simulink model "sim"  (R2024a)
settings: Solver=VariableStepAuto  StartTime=0.0  StopTime=500  RelTol=1e-3
undefined symbols (not defined in the file): K1, K2, K3, Ke1, Ke2, Ke3, Kr
settings Model: Creator=grabo  LastModifiedBy=grabo

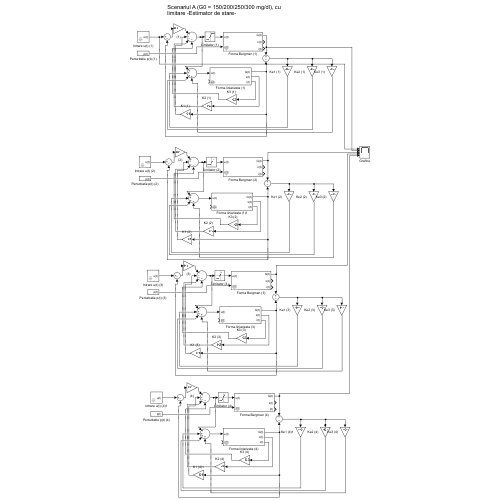
[thumbnail: Simulink's stored preview of the top-level diagram]
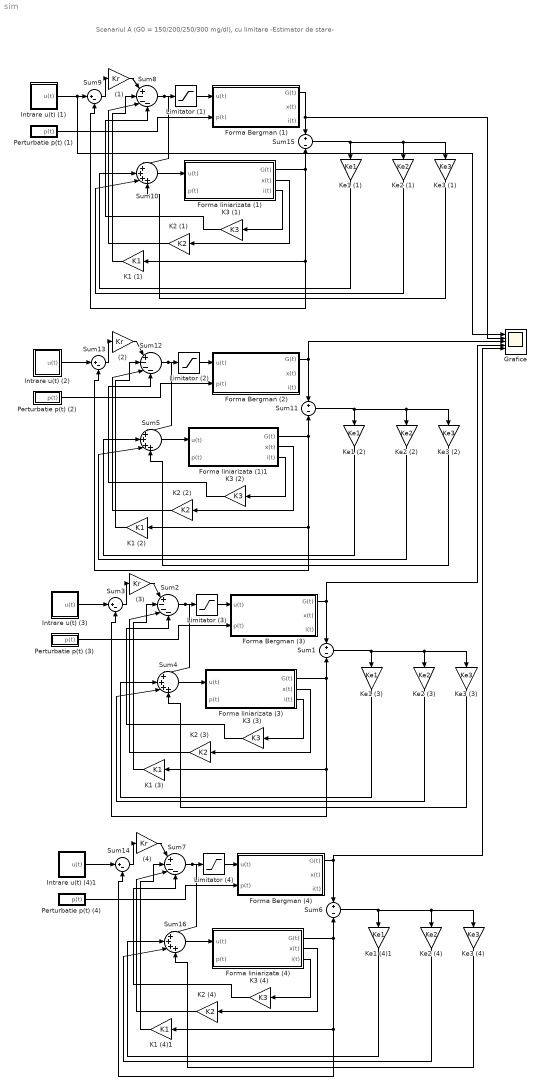
== system sim ==
  note: Scenariul A (G0 = 150/200/250/300 mg/dl), cu limitare -Estimator de stare-
  (1) : Gain  Gain=Kr
  (2) : Gain  Gain=Kr
  (3) : Gain  Gain=Kr
  (4) : Gain  Gain=Kr
  Forma Bergman (1) : Subsystem  mask{V=120, Gb=80, p1=0.019, p2=0.021, p3=10.19*10^(-6), n=0.177, G0=150}
      mask prompts: V "V ="; Gb "Gb ="; p1 "p1 ="; p2 "p2 ="; p3 "p3 ="; n "n ="; G0 "G0 ="
  Forma Bergman (2) : Subsystem  mask{V=120, Gb=80, p1=0.019, p2=0.021, p3=10.19*10^(-6), n=0.177, G0=200}
      mask prompts: V "V ="; Gb "Gb ="; p1 "p1 ="; p2 "p2 ="; p3 "p3 ="; n "n ="; G0 "G0 ="
  Forma Bergman (3) : Subsystem  mask{V=120, Gb=80, p1=0.019, p2=0.021, p3=10.19*10^(-6), n=0.177, G0=250}
      mask prompts: V "V ="; Gb "Gb ="; p1 "p1 ="; p2 "p2 ="; p3 "p3 ="; n "n ="; G0 "G0 ="
  Forma Bergman (4) : Subsystem  mask{V=120, Gb=80, p1=0.019, p2=0.021, p3=10.19*10^(-6), n=0.177, G0=300}
      mask prompts: V "V ="; Gb "Gb ="; p1 "p1 ="; p2 "p2 ="; p3 "p3 ="; n "n ="; G0 "G0 ="
  Forma liniarizata (1) : Subsystem  mask{V=120, Ag=0.8, tgM=40, Xb=0.0054, Gb=80, p1=0.019, p2=0.021, p3=10.19*10^(-6), n=0.177, G0=150}
      mask prompts: V "V ="; Ag "Ag ="; tgM "tgM ="; Xb "Xb ="; Gb "Gb ="; p1 "p1 ="; p2 "p2 ="; p3 "p3 ="; n "n ="; G0 "G0 ="
  Forma liniarizata (1)1 : Subsystem  mask{V=120, Ag=0.8, tgM=40, Xb=0.0054, Gb=80, p1=0.019, p2=0.021, p3=10.19*10^(-6), n=0.177, G0=200}
      mask prompts: V "V ="; Ag "Ag ="; tgM "tgM ="; Xb "Xb ="; Gb "Gb ="; p1 "p1 ="; p2 "p2 ="; p3 "p3 ="; n "n ="; G0 "G0 ="
  Forma liniarizata (3) : Subsystem  mask{V=120, Ag=0.8, tgM=40, Xb=0.0054, Gb=80, p1=0.019, p2=0.021, p3=10.19*10^(-6), n=0.177, G0=250}
      mask prompts: V "V ="; Ag "Ag ="; tgM "tgM ="; Xb "Xb ="; Gb "Gb ="; p1 "p1 ="; p2 "p2 ="; p3 "p3 ="; n "n ="; G0 "G0 ="
  Forma liniarizata (4) : Subsystem  mask{V=120, Ag=0.8, tgM=40, Xb=0.0054, Gb=80, p1=0.019, p2=0.021, p3=10.19*10^(-6), n=0.177, G0=300}
      mask prompts: V "V ="; Ag "Ag ="; tgM "tgM ="; Xb "Xb ="; Gb "Gb ="; p1 "p1 ="; p2 "p2 ="; p3 "p3 ="; n "n ="; G0 "G0 ="
  Grafice : Scope  NumInputPorts=5
  Intrare u(t) (1) : Subsystem  mask{With_u=1, Gref=80}
      mask prompts: With_u "With_u ="; Gref "Gref ="
  Intrare u(t) (2) : Subsystem  mask{With_u=1, Gref=80}
      mask prompts: With_u "With_u ="; Gref "Gref ="
  Intrare u(t) (3) : Subsystem  mask{With_u=1, Gref=80}
      mask prompts: With_u "With_u ="; Gref "Gref ="
  Intrare u(t) (4)1 : Subsystem  mask{With_u=1, Gref=80}
      mask prompts: With_u "With_u ="; Gref "Gref ="
  K1 (1) : Gain  Gain=K1
  K1 (2) : Gain  Gain=K1
  K1 (3) : Gain  Gain=K1
  K1 (4)1 : Gain  Gain=K1
  K2 (1) : Gain  Gain=K2
  K2 (2) : Gain  Gain=K2
  K2 (3) : Gain  Gain=K2
  K2 (4) : Gain  Gain=K2
  K3 (1) : Gain  Gain=K3
  K3 (2) : Gain  Gain=K3
  K3 (3) : Gain  Gain=K3
  K3 (4) : Gain  Gain=K3
  Ke1 (1) : Gain  Gain=Ke1
  Ke1 (2) : Gain  Gain=Ke1
  Ke1 (3) : Gain  Gain=Ke1
  Ke1 (4)1 : Gain  Gain=Ke1
  Ke2 (1) : Gain  Gain=Ke2
  Ke2 (2) : Gain  Gain=Ke2
  Ke2 (3) : Gain  Gain=Ke2
  Ke2 (4) : Gain  Gain=Ke2
  Ke3 (1) : Gain  Gain=Ke3
  Ke3 (2) : Gain  Gain=Ke3
  Ke3 (3) : Gain  Gain=Ke3
  Ke3 (4) : Gain  Gain=Ke3
  Limitator (1) : Saturate  UpperLimit=500  LowerLimit=0
  Limitator (2) : Saturate  UpperLimit=500  LowerLimit=0
  Limitator (3) : Saturate  UpperLimit=500  LowerLimit=0
  Limitator (4) : Saturate  UpperLimit=500  LowerLimit=0
  Perturbatie p(t) (1) : Subsystem  mask{Dg=10*10^3, Ag=0.8, tgM=40, With_p=0}
      mask prompts: Dg "Dg ="; Ag "Ag ="; tgM "tgM ="; With_p "With_p ="
  Perturbatie p(t) (2) : Subsystem  mask{Dg=10*10^3, Ag=0.8, tgM=40, With_p=0}
      mask prompts: Dg "Dg ="; Ag "Ag ="; tgM "tgM ="; With_p "With_p ="
  Perturbatie p(t) (3) : Subsystem  mask{Dg=10*10^3, Ag=0.8, tgM=40, With_p=0}
      mask prompts: Dg "Dg ="; Ag "Ag ="; tgM "tgM ="; With_p "With_p ="
  Perturbatie p(t) (4) : Subsystem  mask{Dg=10*10^3, Ag=0.8, tgM=40, With_p=0}
      mask prompts: Dg "Dg ="; Ag "Ag ="; tgM "tgM ="; With_p "With_p ="
  Sum{1,6,11,15} (4 alike) : Sum  Inputs=+|-
  Sum{4..5,10,16} (4 alike) : Sum  Inputs=|++++
  Sum{2,7..8,12} (4 alike) : Sum  Inputs=|+---
  Sum{3,9,13..14} (4 alike) : Sum  Inputs=|+-
  wires:
  Intrare u(t) (1)/1(u(t)) -> Grafice/1, Sum9/1
  Sum8/1 -> Sum10/1, Limitator (1)/1
  Forma liniarizata (1)/1(G(t)) -> Sum15/2, K1 (1)/1, Sum9/2
  Sum10/1 -> Forma liniarizata (1)/1(u(t))
  Forma liniarizata (1)/2(x(t)) -> K2 (1)/1
  Forma liniarizata (1)/3(i(t)) -> K3 (1)/1
  K1 (1)/1 -> Sum8/2
  K2 (1)/1 -> Sum8/3
  K3 (1)/1 -> Sum8/4
  Sum15/1 -> Ke3 (1)/1, Ke2 (1)/1, Ke1 (1)/1
  Ke1 (1)/1 -> Sum10/2
  Ke2 (1)/1 -> Sum10/3
  Ke3 (1)/1 -> Sum10/4
  Ke1 (2)/1 -> Sum5/2
  Intrare u(t) (2)/1(u(t)) -> Sum13/1
  Sum11/1 -> Ke3 (2)/1, Ke2 (2)/1, Ke1 (2)/1
  K1 (2)/1 -> Sum12/2
  K2 (2)/1 -> Sum12/3
  Forma liniarizata (1)1/1(G(t)) -> Sum11/2, K1 (2)/1, Sum13/2
  Sum5/1 -> Forma liniarizata (1)1/1(u(t))
  Sum12/1 -> Sum5/1, Limitator (2)/1
  K3 (2)/1 -> Sum12/4
  Ke3 (2)/1 -> Sum5/4
  Forma Bergman (2)/1(G(t)) -> Grafice/3, Sum11/1
  Forma liniarizata (1)1/2(x(t)) -> K2 (2)/1
  Forma liniarizata (1)1/3(i(t)) -> K3 (2)/1
  Ke2 (2)/1 -> Sum5/3
  (1)/1 -> Sum8/1
  Sum9/1 -> (1)/1
  (2)/1 -> Sum12/1
  Sum13/1 -> (2)/1
  Forma Bergman (1)/1(G(t)) -> Grafice/2, Sum15/1
  Limitator (2)/1 -> Forma Bergman (2)/1(u(t))
  Limitator (1)/1 -> Forma Bergman (1)/1(u(t))
  Perturbatie p(t) (1)/1(p(t)) -> Forma Bergman (1)/2(p(t))
  Perturbatie p(t) (2)/1(p(t)) -> Forma Bergman (2)/2(p(t))
  Perturbatie p(t) (3)/1(p(t)) -> Forma Bergman (3)/2(p(t))
  Limitator (3)/1 -> Forma Bergman (3)/1(u(t))
  Ke1 (3)/1 -> Sum4/2
  Ke2 (3)/1 -> Sum4/3
  K3 (3)/1 -> Sum2/4
  Forma liniarizata (3)/1(G(t)) -> Sum1/2, K1 (3)/1, Sum3/2
  Forma Bergman (3)/1(G(t)) -> Grafice/4, Sum1/1
  Ke3 (3)/1 -> Sum4/4
  Sum2/1 -> Sum4/1, Limitator (3)/1
  Forma liniarizata (3)/3(i(t)) -> K3 (3)/1
  Sum4/1 -> Forma liniarizata (3)/1(u(t))
  K2 (3)/1 -> Sum2/3
  K1 (3)/1 -> Sum2/2
  (3)/1 -> Sum2/1
  Intrare u(t) (3)/1(u(t)) -> Sum3/1
  Forma liniarizata (3)/2(x(t)) -> K2 (3)/1
  Sum1/1 -> Ke3 (3)/1, Ke2 (3)/1, Ke1 (3)/1
  Sum3/1 -> (3)/1
  Perturbatie p(t) (4)/1(p(t)) -> Forma Bergman (4)/2(p(t))
  Limitator (4)/1 -> Forma Bergman (4)/1(u(t))
  Ke1 (4)1/1 -> Sum16/2
  Ke2 (4)/1 -> Sum16/3
  K3 (4)/1 -> Sum7/4
  Forma liniarizata (4)/1(G(t)) -> Sum6/2, K1 (4)1/1, Sum14/2
  Forma Bergman (4)/1(G(t)) -> Grafice/5, Sum6/1
  Ke3 (4)/1 -> Sum16/4
  Sum7/1 -> Sum16/1, Limitator (4)/1
  Forma liniarizata (4)/3(i(t)) -> K3 (4)/1
  Sum16/1 -> Forma liniarizata (4)/1(u(t))
  K2 (4)/1 -> Sum7/3
  K1 (4)1/1 -> Sum7/2
  (4)/1 -> Sum7/1
  Intrare u(t) (4)1/1(u(t)) -> Sum14/1
  Forma liniarizata (4)/2(x(t)) -> K2 (4)/1
  Sum6/1 -> Ke3 (4)/1, Ke2 (4)/1, Ke1 (4)1/1
  Sum14/1 -> (4)/1

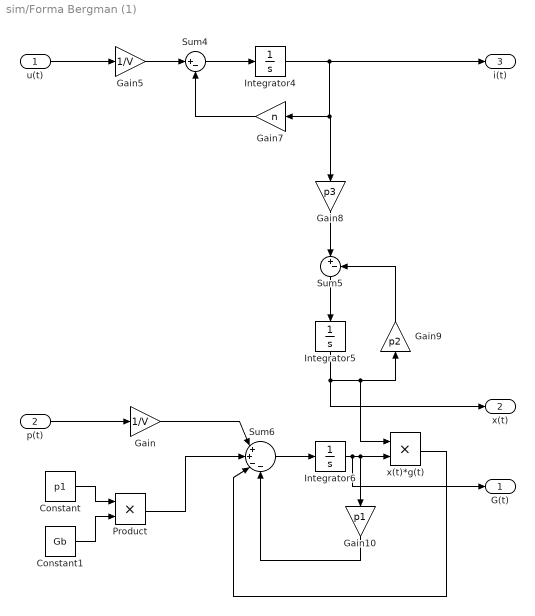
== system sim/Forma Bergman (1) ==
  u(t) : Inport
  p(t) : Inport  Port=2
  Constant : Constant  Value=p1
  Constant1 : Constant  Value=Gb
  Gain : Gain  Gain=1/V
  Gain10 : Gain  Gain=p1
  Gain5 : Gain  Gain=1/V
  Gain7 : Gain  Gain=n
  Gain8 : Gain  Gain=p3
  Gain9 : Gain  Gain=p2
  Integrator4 : Integrator
  Integrator5 : Integrator
  Integrator6 : Integrator  InitialCondition=G0
  Product : Product
  Sum4 : Sum  Inputs=|+-
  Sum5 : Sum  Inputs=|+-
  Sum6 : Sum  Inputs=|++--
  x(t)*g(t) : Product
  G(t) : Outport
  x(t) : Outport  Port=2
  i(t) : Outport  Port=3
  wires:
  Sum4/1 -> Integrator4/1
  Gain7/1 -> Sum4/2
  Integrator4/1 -> Gain7/1, Gain8/1, i(t)/1
  Gain8/1 -> Sum5/1
  Sum5/1 -> Integrator5/1
  Gain9/1 -> Sum5/2
  Sum6/1 -> Integrator6/1
  Integrator6/1 -> G(t)/1, Gain10/1, x(t)*g(t)/2
  Gain10/1 -> Sum6/4
  x(t)*g(t)/1 -> Sum6/3
  Product/1 -> Sum6/2
  Integrator5/1 -> x(t)/1, x(t)*g(t)/1, Gain9/1
  Gain5/1 -> Sum4/1
  u(t)/1 -> Gain5/1
  p(t)/1 -> Gain/1
  Gain/1 -> Sum6/1
  Constant/1 -> Product/1
  Constant1/1 -> Product/2

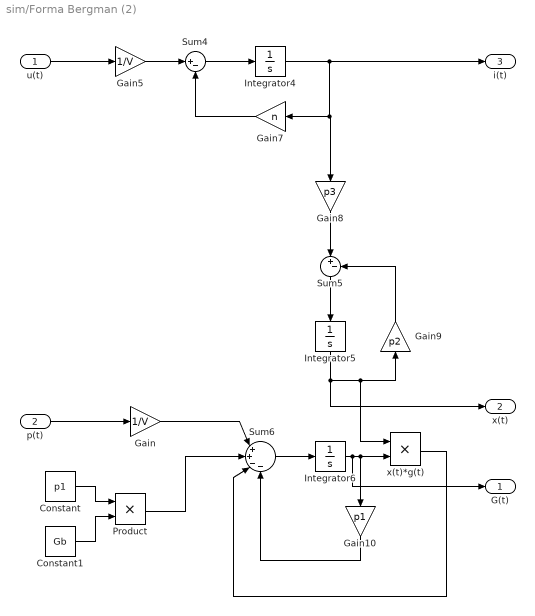
== system sim/Forma Bergman (2) ==
  u(t) : Inport
  p(t) : Inport  Port=2
  Constant : Constant  Value=p1
  Constant1 : Constant  Value=Gb
  Gain : Gain  Gain=1/V
  Gain10 : Gain  Gain=p1
  Gain5 : Gain  Gain=1/V
  Gain7 : Gain  Gain=n
  Gain8 : Gain  Gain=p3
  Gain9 : Gain  Gain=p2
  Integrator4 : Integrator
  Integrator5 : Integrator
  Integrator6 : Integrator  InitialCondition=G0
  Product : Product
  Sum4 : Sum  Inputs=|+-
  Sum5 : Sum  Inputs=|+-
  Sum6 : Sum  Inputs=|++--
  x(t)*g(t) : Product
  G(t) : Outport
  x(t) : Outport  Port=2
  i(t) : Outport  Port=3
  wires:
  Sum4/1 -> Integrator4/1
  Gain7/1 -> Sum4/2
  Integrator4/1 -> Gain7/1, Gain8/1, i(t)/1
  Gain8/1 -> Sum5/1
  Sum5/1 -> Integrator5/1
  Gain9/1 -> Sum5/2
  Sum6/1 -> Integrator6/1
  Integrator6/1 -> G(t)/1, Gain10/1, x(t)*g(t)/2
  Gain10/1 -> Sum6/4
  x(t)*g(t)/1 -> Sum6/3
  Product/1 -> Sum6/2
  Integrator5/1 -> x(t)/1, x(t)*g(t)/1, Gain9/1
  Gain5/1 -> Sum4/1
  u(t)/1 -> Gain5/1
  p(t)/1 -> Gain/1
  Gain/1 -> Sum6/1
  Constant/1 -> Product/1
  Constant1/1 -> Product/2

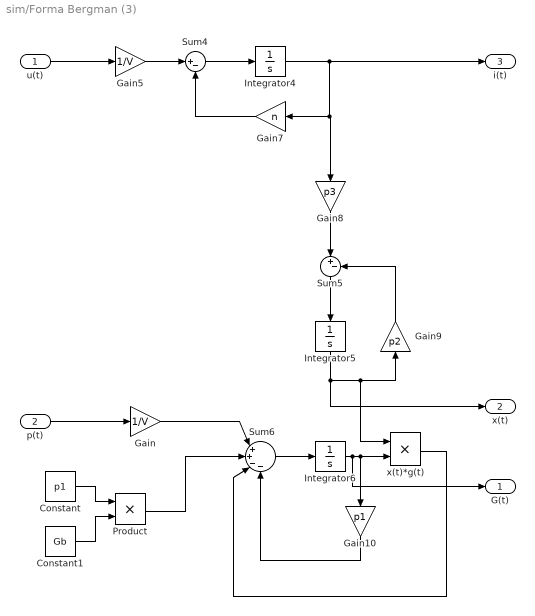
== system sim/Forma Bergman (3) ==
  u(t) : Inport
  p(t) : Inport  Port=2
  Constant : Constant  Value=p1
  Constant1 : Constant  Value=Gb
  Gain : Gain  Gain=1/V
  Gain10 : Gain  Gain=p1
  Gain5 : Gain  Gain=1/V
  Gain7 : Gain  Gain=n
  Gain8 : Gain  Gain=p3
  Gain9 : Gain  Gain=p2
  Integrator4 : Integrator
  Integrator5 : Integrator
  Integrator6 : Integrator  InitialCondition=G0
  Product : Product
  Sum4 : Sum  Inputs=|+-
  Sum5 : Sum  Inputs=|+-
  Sum6 : Sum  Inputs=|++--
  x(t)*g(t) : Product
  G(t) : Outport
  x(t) : Outport  Port=2
  i(t) : Outport  Port=3
  wires:
  Sum4/1 -> Integrator4/1
  Gain7/1 -> Sum4/2
  Integrator4/1 -> Gain7/1, Gain8/1, i(t)/1
  Gain8/1 -> Sum5/1
  Sum5/1 -> Integrator5/1
  Gain9/1 -> Sum5/2
  Sum6/1 -> Integrator6/1
  Integrator6/1 -> G(t)/1, Gain10/1, x(t)*g(t)/2
  Gain10/1 -> Sum6/4
  x(t)*g(t)/1 -> Sum6/3
  Product/1 -> Sum6/2
  Integrator5/1 -> x(t)/1, x(t)*g(t)/1, Gain9/1
  Gain5/1 -> Sum4/1
  u(t)/1 -> Gain5/1
  p(t)/1 -> Gain/1
  Gain/1 -> Sum6/1
  Constant/1 -> Product/1
  Constant1/1 -> Product/2

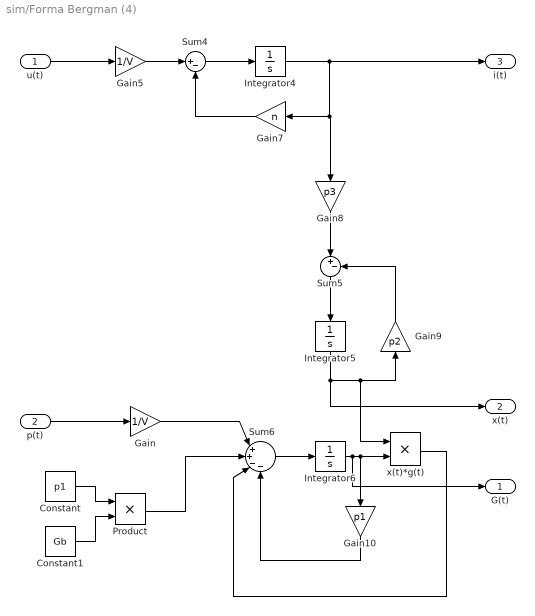
== system sim/Forma Bergman (4) ==
  u(t) : Inport
  p(t) : Inport  Port=2
  Constant : Constant  Value=p1
  Constant1 : Constant  Value=Gb
  Gain : Gain  Gain=1/V
  Gain10 : Gain  Gain=p1
  Gain5 : Gain  Gain=1/V
  Gain7 : Gain  Gain=n
  Gain8 : Gain  Gain=p3
  Gain9 : Gain  Gain=p2
  Integrator4 : Integrator
  Integrator5 : Integrator
  Integrator6 : Integrator  InitialCondition=G0
  Product : Product
  Sum4 : Sum  Inputs=|+-
  Sum5 : Sum  Inputs=|+-
  Sum6 : Sum  Inputs=|++--
  x(t)*g(t) : Product
  G(t) : Outport
  x(t) : Outport  Port=2
  i(t) : Outport  Port=3
  wires:
  Sum4/1 -> Integrator4/1
  Gain7/1 -> Sum4/2
  Integrator4/1 -> Gain7/1, Gain8/1, i(t)/1
  Gain8/1 -> Sum5/1
  Sum5/1 -> Integrator5/1
  Gain9/1 -> Sum5/2
  Sum6/1 -> Integrator6/1
  Integrator6/1 -> G(t)/1, Gain10/1, x(t)*g(t)/2
  Gain10/1 -> Sum6/4
  x(t)*g(t)/1 -> Sum6/3
  Product/1 -> Sum6/2
  Integrator5/1 -> x(t)/1, x(t)*g(t)/1, Gain9/1
  Gain5/1 -> Sum4/1
  u(t)/1 -> Gain5/1
  p(t)/1 -> Gain/1
  Gain/1 -> Sum6/1
  Constant/1 -> Product/1
  Constant1/1 -> Product/2

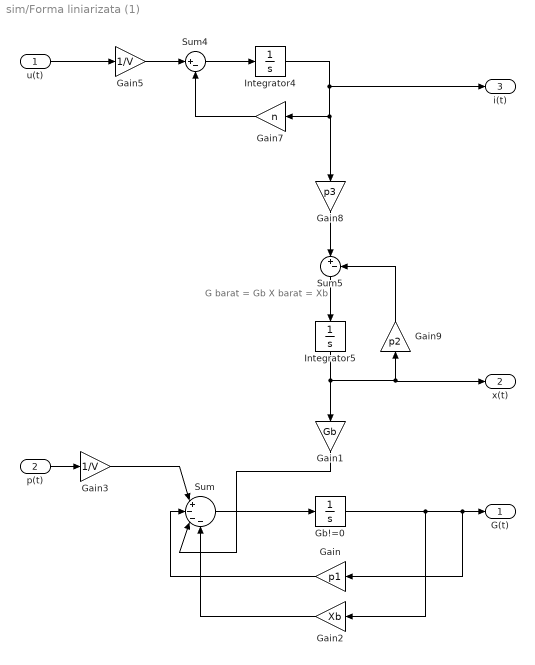
== system sim/Forma liniarizata (1) ==
  note: G barat = Gb
      | X barat = Xb
  u(t) : Inport
  p(t) : Inport  Port=2
  Gain : Gain  Gain=p1
  Gain1 : Gain  Gain=Gb
  Gain2 : Gain  Gain=Xb
  Gain3 : Gain  Gain=1/V
  Gain5 : Gain  Gain=1/V
  Gain7 : Gain  Gain=n
  Gain8 : Gain  Gain=p3
  Gain9 : Gain  Gain=p2
  Gb!=0 : Integrator  InitialCondition=G0
  Integrator4 : Integrator
  Integrator5 : Integrator
  Sum : Sum  Inputs=|+---
  Sum4 : Sum  Inputs=|+-
  Sum5 : Sum  Inputs=|+-
  G(t) : Outport
  x(t) : Outport  Port=2
  i(t) : Outport  Port=3
  wires:
  Sum4/1 -> Integrator4/1
  Gain7/1 -> Sum4/2
  Integrator4/1 -> i(t)/1, Gain7/1, Gain8/1
  Gain8/1 -> Sum5/1
  Sum5/1 -> Integrator5/1
  Gain9/1 -> Sum5/2
  Integrator5/1 -> Gain1/1, Gain9/1, x(t)/1
  Gain5/1 -> Sum4/1
  u(t)/1 -> Gain5/1
  Sum/1 -> Gb!=0/1
  Gain/1 -> Sum/2
  Gb!=0/1 -> Gain2/1, G(t)/1, Gain/1
  Gain1/1 -> Sum/3
  Gain2/1 -> Sum/4
  p(t)/1 -> Gain3/1
  Gain3/1 -> Sum/1

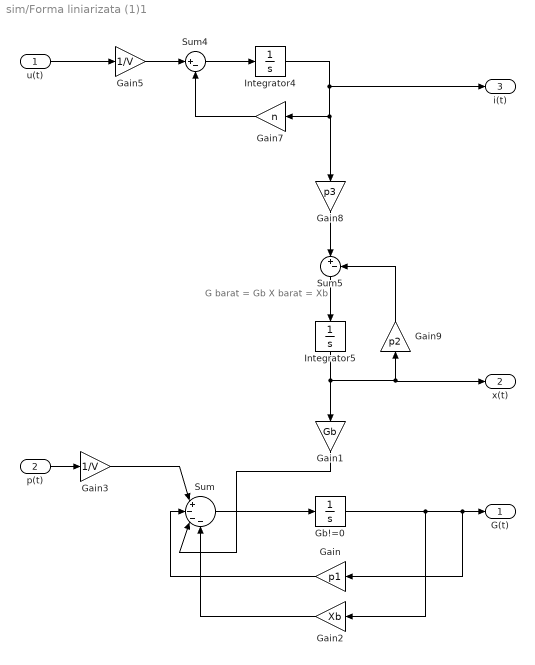
== system sim/Forma liniarizata (1)1 ==
  note: G barat = Gb
      | X barat = Xb
  u(t) : Inport
  p(t) : Inport  Port=2
  Gain : Gain  Gain=p1
  Gain1 : Gain  Gain=Gb
  Gain2 : Gain  Gain=Xb
  Gain3 : Gain  Gain=1/V
  Gain5 : Gain  Gain=1/V
  Gain7 : Gain  Gain=n
  Gain8 : Gain  Gain=p3
  Gain9 : Gain  Gain=p2
  Gb!=0 : Integrator  InitialCondition=G0
  Integrator4 : Integrator
  Integrator5 : Integrator
  Sum : Sum  Inputs=|+---
  Sum4 : Sum  Inputs=|+-
  Sum5 : Sum  Inputs=|+-
  G(t) : Outport
  x(t) : Outport  Port=2
  i(t) : Outport  Port=3
  wires:
  Sum4/1 -> Integrator4/1
  Gain7/1 -> Sum4/2
  Integrator4/1 -> i(t)/1, Gain7/1, Gain8/1
  Gain8/1 -> Sum5/1
  Sum5/1 -> Integrator5/1
  Gain9/1 -> Sum5/2
  Integrator5/1 -> Gain1/1, Gain9/1, x(t)/1
  Gain5/1 -> Sum4/1
  u(t)/1 -> Gain5/1
  Sum/1 -> Gb!=0/1
  Gain/1 -> Sum/2
  Gb!=0/1 -> Gain2/1, G(t)/1, Gain/1
  Gain1/1 -> Sum/3
  Gain2/1 -> Sum/4
  p(t)/1 -> Gain3/1
  Gain3/1 -> Sum/1

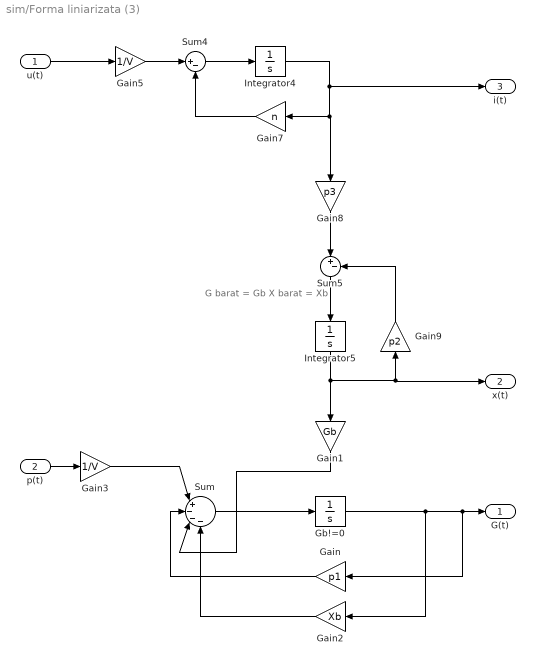
== system sim/Forma liniarizata (3) ==
  note: G barat = Gb
      | X barat = Xb
  u(t) : Inport
  p(t) : Inport  Port=2
  Gain : Gain  Gain=p1
  Gain1 : Gain  Gain=Gb
  Gain2 : Gain  Gain=Xb
  Gain3 : Gain  Gain=1/V
  Gain5 : Gain  Gain=1/V
  Gain7 : Gain  Gain=n
  Gain8 : Gain  Gain=p3
  Gain9 : Gain  Gain=p2
  Gb!=0 : Integrator  InitialCondition=G0
  Integrator4 : Integrator
  Integrator5 : Integrator
  Sum : Sum  Inputs=|+---
  Sum4 : Sum  Inputs=|+-
  Sum5 : Sum  Inputs=|+-
  G(t) : Outport
  x(t) : Outport  Port=2
  i(t) : Outport  Port=3
  wires:
  Sum4/1 -> Integrator4/1
  Gain7/1 -> Sum4/2
  Integrator4/1 -> i(t)/1, Gain7/1, Gain8/1
  Gain8/1 -> Sum5/1
  Sum5/1 -> Integrator5/1
  Gain9/1 -> Sum5/2
  Integrator5/1 -> Gain1/1, Gain9/1, x(t)/1
  Gain5/1 -> Sum4/1
  u(t)/1 -> Gain5/1
  Sum/1 -> Gb!=0/1
  Gain/1 -> Sum/2
  Gb!=0/1 -> Gain2/1, G(t)/1, Gain/1
  Gain1/1 -> Sum/3
  Gain2/1 -> Sum/4
  p(t)/1 -> Gain3/1
  Gain3/1 -> Sum/1

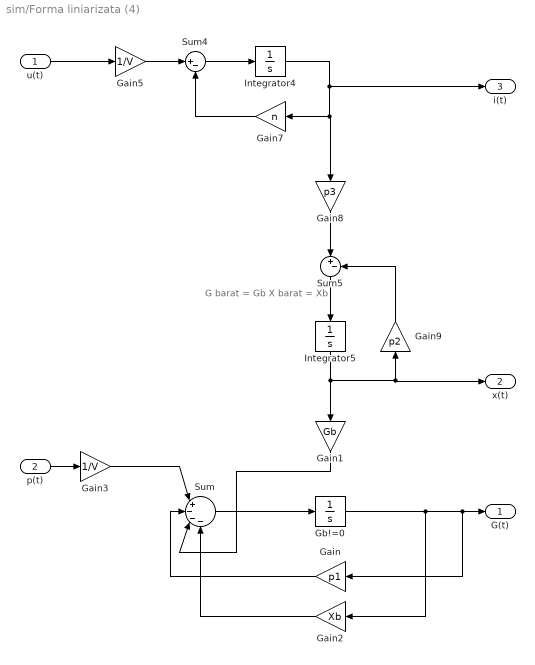
== system sim/Forma liniarizata (4) ==
  note: G barat = Gb
      | X barat = Xb
  u(t) : Inport
  p(t) : Inport  Port=2
  Gain : Gain  Gain=p1
  Gain1 : Gain  Gain=Gb
  Gain2 : Gain  Gain=Xb
  Gain3 : Gain  Gain=1/V
  Gain5 : Gain  Gain=1/V
  Gain7 : Gain  Gain=n
  Gain8 : Gain  Gain=p3
  Gain9 : Gain  Gain=p2
  Gb!=0 : Integrator  InitialCondition=G0
  Integrator4 : Integrator
  Integrator5 : Integrator
  Sum : Sum  Inputs=|+---
  Sum4 : Sum  Inputs=|+-
  Sum5 : Sum  Inputs=|+-
  G(t) : Outport
  x(t) : Outport  Port=2
  i(t) : Outport  Port=3
  wires:
  Sum4/1 -> Integrator4/1
  Gain7/1 -> Sum4/2
  Integrator4/1 -> i(t)/1, Gain7/1, Gain8/1
  Gain8/1 -> Sum5/1
  Sum5/1 -> Integrator5/1
  Gain9/1 -> Sum5/2
  Integrator5/1 -> Gain1/1, Gain9/1, x(t)/1
  Gain5/1 -> Sum4/1
  u(t)/1 -> Gain5/1
  Sum/1 -> Gb!=0/1
  Gain/1 -> Sum/2
  Gb!=0/1 -> Gain2/1, G(t)/1, Gain/1
  Gain1/1 -> Sum/3
  Gain2/1 -> Sum/4
  p(t)/1 -> Gain3/1
  Gain3/1 -> Sum/1

== system sim/Intrare u(t) (1) ==
  Gain : Gain  Gain=With_u
  Step : Step  Time=0  After=Gref  SampleTime=0
  u(t) : Outport
  wires:
  Step/1 -> Gain/1
  Gain/1 -> u(t)/1

== system sim/Intrare u(t) (2) ==
  Gain : Gain  Gain=With_u
  Step : Step  Time=0  After=Gref  SampleTime=0
  u(t) : Outport
  wires:
  Step/1 -> Gain/1
  Gain/1 -> u(t)/1

== system sim/Intrare u(t) (3) ==
  Gain : Gain  Gain=With_u
  Step : Step  Time=0  After=Gref  SampleTime=0
  u(t) : Outport
  wires:
  Step/1 -> Gain/1
  Gain/1 -> u(t)/1

== system sim/Intrare u(t) (4)1 ==
  Gain : Gain  Gain=With_u
  Step : Step  Time=0  After=Gref  SampleTime=0
  u(t) : Outport
  wires:
  Step/1 -> Gain/1
  Gain/1 -> u(t)/1

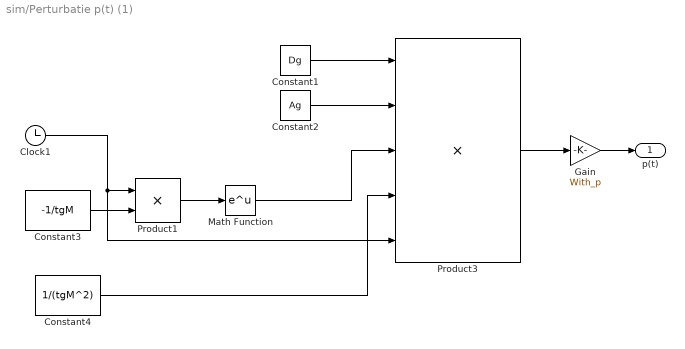
== system sim/Perturbatie p(t) (1) ==
  Clock1 : Clock
  Constant1 : Constant  Value=Dg
  Constant2 : Constant  Value=Ag
  Constant3 : Constant  Value=-1/tgM
  Constant4 : Constant  Value=1/(tgM^2)
  Gain : Gain  Gain=With_p
  Math Function : Math  SignedPower=on
  Product1 : Product
  Product3 : Product  Inputs=5
  p(t) : Outport
  wires:
  Clock1/1 -> Product3/5, Product1/1
  Constant3/1 -> Product1/2
  Product1/1 -> Math Function/1
  Constant4/1 -> Product3/4
  Constant1/1 -> Product3/1
  Constant2/1 -> Product3/2
  Math Function/1 -> Product3/3
  Product3/1 -> Gain/1
  Gain/1 -> p(t)/1

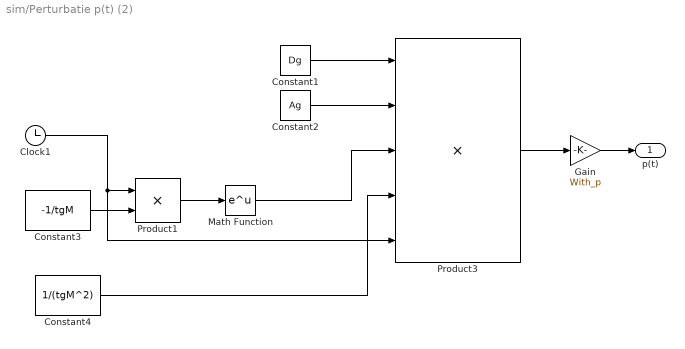
== system sim/Perturbatie p(t) (2) ==
  Clock1 : Clock
  Constant1 : Constant  Value=Dg
  Constant2 : Constant  Value=Ag
  Constant3 : Constant  Value=-1/tgM
  Constant4 : Constant  Value=1/(tgM^2)
  Gain : Gain  Gain=With_p
  Math Function : Math  SignedPower=on
  Product1 : Product
  Product3 : Product  Inputs=5
  p(t) : Outport
  wires:
  Clock1/1 -> Product3/5, Product1/1
  Constant3/1 -> Product1/2
  Product1/1 -> Math Function/1
  Constant4/1 -> Product3/4
  Constant1/1 -> Product3/1
  Constant2/1 -> Product3/2
  Math Function/1 -> Product3/3
  Product3/1 -> Gain/1
  Gain/1 -> p(t)/1

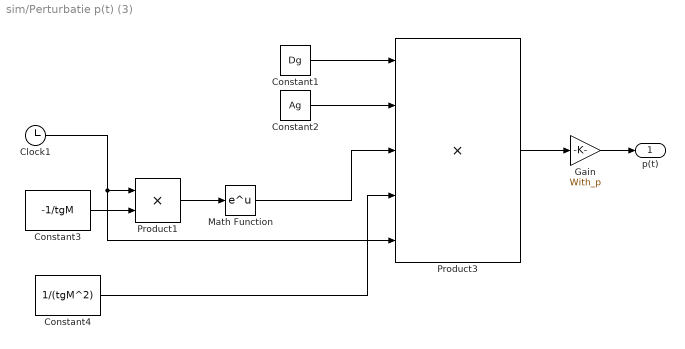
== system sim/Perturbatie p(t) (3) ==
  Clock1 : Clock
  Constant1 : Constant  Value=Dg
  Constant2 : Constant  Value=Ag
  Constant3 : Constant  Value=-1/tgM
  Constant4 : Constant  Value=1/(tgM^2)
  Gain : Gain  Gain=With_p
  Math Function : Math  SignedPower=on
  Product1 : Product
  Product3 : Product  Inputs=5
  p(t) : Outport
  wires:
  Clock1/1 -> Product3/5, Product1/1
  Constant3/1 -> Product1/2
  Product1/1 -> Math Function/1
  Constant4/1 -> Product3/4
  Constant1/1 -> Product3/1
  Constant2/1 -> Product3/2
  Math Function/1 -> Product3/3
  Product3/1 -> Gain/1
  Gain/1 -> p(t)/1

== system sim/Perturbatie p(t) (4) ==
  Clock1 : Clock
  Constant1 : Constant  Value=Dg
  Constant2 : Constant  Value=Ag
  Constant3 : Constant  Value=-1/tgM
  Constant4 : Constant  Value=1/(tgM^2)
  Gain : Gain  Gain=With_p
  Math Function : Math  SignedPower=on
  Product1 : Product
  Product3 : Product  Inputs=5
  p(t) : Outport
  wires:
  Clock1/1 -> Product3/5, Product1/1
  Constant3/1 -> Product1/2
  Product1/1 -> Math Function/1
  Constant4/1 -> Product3/4
  Constant1/1 -> Product3/1
  Constant2/1 -> Product3/2
  Math Function/1 -> Product3/3
  Product3/1 -> Gain/1
  Gain/1 -> p(t)/1
